simulink model "unicycle"  (R2024a)
settings: Solver=ode45  StartTime=0.0  StopTime=20.0  RelTol=1e-3
undefined symbols (not defined in the file): b_reference_point, damping_coefficient, damping_coefficient_nl, k1, k2, kp1, kp2, kp3, kp4, kv, kw, natural_frequency, natural_frequency_nl, radius, x1_dest, x2_dest, x3_dest
libraries: simulink x6, robotmobilelib x3
(part 1 of 2)
settings Model: Creator=leona  LastModifiedBy=meteh
settings SolverCC: ZeroCrossAlgorithm=Adaptive
settings DataIOCC: SaveFinalState=on  SaveFormat=StructureWithTime  SaveState=on  SignalLogging=off
settings DebuggingCC: IgnoredZcDiagnostic=none

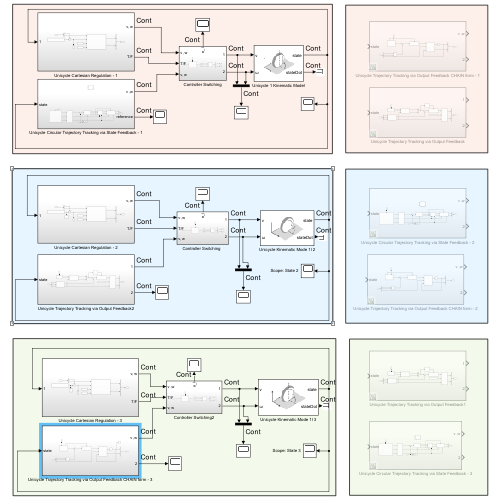
[thumbnail: Simulink's stored preview of the top-level diagram]
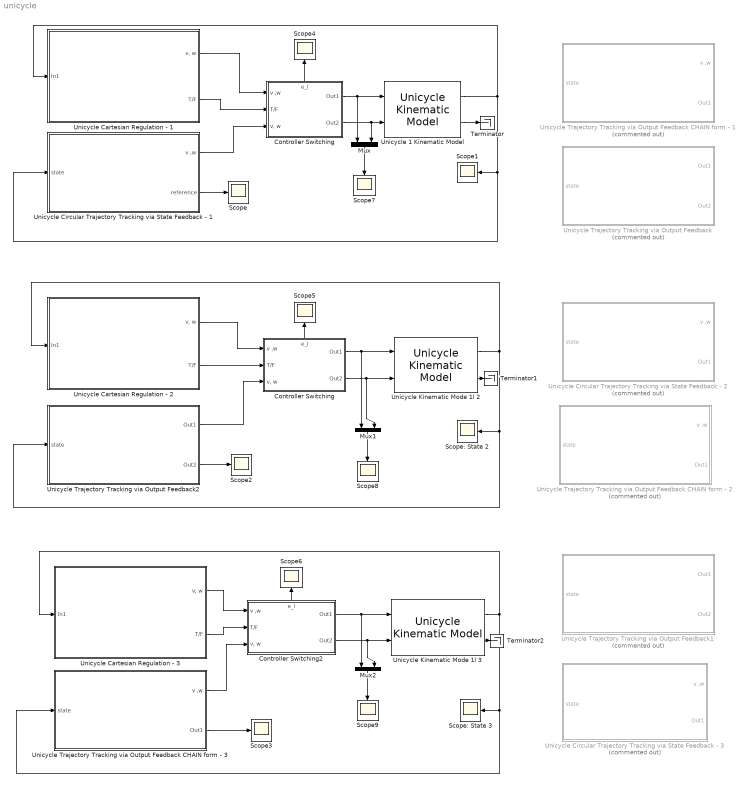
== system unicycle ==
  Controller Switching : Subsystem
      settings: PortSchema="{\"entries\":[{\"content\":{\"sides\":[{\"content\":{\"connectorIds\":[\"In1\",\"In2\",\"In3\"]},\"type\":\"ConnectorPlacement.EquallySpacedRectSide\",\"uuid\":\"584f21ea-dfd6-45f5-be40-b293bc8457b1\"},{\"content\":{\"connectorIds\":[\"Out1\",\"Out2\"],\"side\":\"RIGHT\"},\"type\":\"ConnectorPlacement.EquallySpacedRectSide\",\"uuid\":\"f9bf7ef9-3ae2-4892-b478-b0129d05cdbd\"},{\"content\":{\"connectorIds\":[\"Out3\"],\"side\":\"TOP\"},\"type\":\"ConnectorPlacement.EquallySpacedRectSide\",\"uuid\":\"62fa3bd1-cc21-4bdf-9148-7b9ede413ebd\"}]},\"type\":\"ConnectorPlacement.EquallySpacedConnector\",\"uuid\":\"adaa0c4e-8ae6-4cf2-baff-ed3c22a40f8d\"}],\"packageUris\":[\"http://schema.mathworks.com/mf0/Connector/R2020b\"],\"version\":\"1.0\"}"
  "Controller Switching  " : Subsystem
      settings: PortSchema="{\"entries\":[{\"content\":{\"sides\":[{\"content\":{\"connectorIds\":[\"In1\",\"In2\",\"In3\"]},\"type\":\"ConnectorPlacement.EquallySpacedRectSide\",\"uuid\":\"584f21ea-dfd6-45f5-be40-b293bc8457b1\"},{\"content\":{\"connectorIds\":[\"Out1\",\"Out2\"],\"side\":\"RIGHT\"},\"type\":\"ConnectorPlacement.EquallySpacedRectSide\",\"uuid\":\"f9bf7ef9-3ae2-4892-b478-b0129d05cdbd\"},{\"content\":{\"connectorIds\":[\"Out3\"],\"side\":\"TOP\"},\"type\":\"ConnectorPlacement.EquallySpacedRectSide\",\"uuid\":\"62fa3bd1-cc21-4bdf-9148-7b9ede413ebd\"}]},\"type\":\"ConnectorPlacement.EquallySpacedConnector\",\"uuid\":\"adaa0c4e-8ae6-4cf2-baff-ed3c22a40f8d\"}],\"packageUris\":[\"http://schema.mathworks.com/mf0/Connector/R2020b\"],\"version\":\"1.0\"}"
  Controller Switching2 : Subsystem
      settings: PortSchema="{\"entries\":[{\"content\":{\"sides\":[{\"content\":{\"connectorIds\":[\"In1\",\"In2\",\"In3\"]},\"type\":\"ConnectorPlacement.EquallySpacedRectSide\",\"uuid\":\"584f21ea-dfd6-45f5-be40-b293bc8457b1\"},{\"content\":{\"connectorIds\":[\"Out1\",\"Out2\"],\"side\":\"RIGHT\"},\"type\":\"ConnectorPlacement.EquallySpacedRectSide\",\"uuid\":\"f9bf7ef9-3ae2-4892-b478-b0129d05cdbd\"},{\"content\":{\"connectorIds\":[\"Out3\"],\"side\":\"TOP\"},\"type\":\"ConnectorPlacement.EquallySpacedRectSide\",\"uuid\":\"62fa3bd1-cc21-4bdf-9148-7b9ede413ebd\"}]},\"type\":\"ConnectorPlacement.EquallySpacedConnector\",\"uuid\":\"adaa0c4e-8ae6-4cf2-baff-ed3c22a40f8d\"}],\"packageUris\":[\"http://schema.mathworks.com/mf0/Connector/R2020b\"],\"version\":\"1.0\"}"
  Mux : Mux  Inputs=2
  Mux1 : Mux  Inputs=2
  Mux2 : Mux  Inputs=2
  Scope{,1..9} (10 alike) : Scope
  Scope: State 2 : Scope
  Scope: State 3 : Scope
  Terminator : Terminator
  Terminator1 : Terminator
  Terminator2 : Terminator
  Unicycle 1 Kinematic Model : robotmobilelib/Unicycle Kinematic Model  VehicleInputs=Vehicle Speed & Heading Angular Velocity  WheelRadius=wheel_radius  WheelSpeedRange=wheel_speed_range  InitialState=init_state_1  SimulateUsing=Interpreted execution
  Unicycle Cartesian Regulation - 1 : Subsystem
  Unicycle Cartesian Regulation - 2 : Subsystem
  Unicycle Cartesian Regulation - 3 : Subsystem
  Unicycle Circular Trajectory Tracking via State Feedback - 1 : Subsystem
  Unicycle Circular Trajectory Tracking via State Feedback - 2 : Subsystem  Commented=on
  Unicycle Circular Trajectory Tracking via State Feedback - 3 : Subsystem  Commented=on
  Unicycle Kinematic Mode 1l 2 : robotmobilelib/Unicycle Kinematic Model  VehicleInputs=Vehicle Speed & Heading Angular Velocity  WheelRadius=wheel_radius  WheelSpeedRange=wheel_speed_range  InitialState=init_state_2  SimulateUsing=Interpreted execution
  Unicycle Kinematic Mode 1l 3 : robotmobilelib/Unicycle Kinematic Model  VehicleInputs=Vehicle Speed & Heading Angular Velocity  WheelRadius=wheel_radius  WheelSpeedRange=wheel_speed_range  InitialState=init_state_3  SimulateUsing=Interpreted execution
  Unicycle Trajectory Tracking via Output Feedback : Subsystem  Commented=on
  Unicycle Trajectory Tracking via Output Feedback CHAIN form - 1 : Subsystem  Commented=on
  Unicycle Trajectory Tracking via Output Feedback CHAIN form - 2 : Subsystem  Commented=on
  Unicycle Trajectory Tracking via Output Feedback CHAIN form - 3 : Subsystem
  Unicycle Trajectory Tracking via Output Feedback1 : Subsystem  Commented=on
  Unicycle Trajectory Tracking via Output Feedback2 : Subsystem
  wires:
  Unicycle Cartesian Regulation - 1/1("v, w") -> Controller Switching/1(v ,w)
  Controller Switching/2(Out2) -> Mux/2, Unicycle 1 Kinematic Model/2
  Controller Switching/1(Out1) -> Unicycle 1 Kinematic Model/1, Mux/1
  Unicycle 1 Kinematic Model/1 -> Unicycle Cartesian Regulation - 1/1(In1), Unicycle Circular Trajectory Tracking via State Feedback - 1/1("state "), Scope1/1
  Unicycle Circular Trajectory Tracking via State Feedback - 1/1(v ,w) -> Controller Switching/3("v, w")
  Unicycle Cartesian Regulation - 1/2(T/F) -> Controller Switching/2(T/F)
  Unicycle Cartesian Regulation - 2/1("v, w") -> "Controller Switching  "/1(v ,w)
  Unicycle Cartesian Regulation - 2/2(T/F) -> "Controller Switching  "/2(T/F)
  Unicycle Trajectory Tracking via Output Feedback2/1(Out1) -> "Controller Switching  "/3("v, w")
  Unicycle Kinematic Mode 1l 2/2 -> Terminator1/1
  Unicycle Kinematic Mode 1l 2/1 -> Unicycle Cartesian Regulation - 2/1(In1), Unicycle Trajectory Tracking via Output Feedback2/1(state), Scope: State 2/1
  Controller Switching2/2(Out2) -> Unicycle Kinematic Mode 1l 3/2, Mux2/2
  Unicycle Kinematic Mode 1l 3/2 -> Terminator2/1
  Unicycle Kinematic Mode 1l 3/1 -> Unicycle Cartesian Regulation - 3/1(In1), Unicycle Trajectory Tracking via Output Feedback CHAIN form - 3/1(state), Scope: State 3/1
  Controller Switching2/1(Out1) -> Mux2/1, Unicycle Kinematic Mode 1l 3/1
  Unicycle 1 Kinematic Model/2 -> Terminator/1
  Unicycle Cartesian Regulation - 3/1("v, w") -> Controller Switching2/1(v ,w)
  Unicycle Cartesian Regulation - 3/2(T/F) -> Controller Switching2/2(T/F)
  Unicycle Trajectory Tracking via Output Feedback CHAIN form - 3/1(v ,w) -> Controller Switching2/3("v, w")
  Unicycle Circular Trajectory Tracking via State Feedback - 1/2(reference) -> Scope/1
  Unicycle Trajectory Tracking via Output Feedback2/2(Out2) -> Scope2/1
  Unicycle Trajectory Tracking via Output Feedback CHAIN form - 3/2(Out1) -> Scope3/1
  Controller Switching/3(e_l) -> Scope4/1
  "Controller Switching  "/3(e_l) -> Scope5/1
  Controller Switching2/3(e_l) -> Scope6/1
  Mux/1 -> Scope7/1
  Mux1/1 -> Scope8/1
  Mux2/1 -> Scope9/1
  "Controller Switching  "/1(Out1) -> Unicycle Kinematic Mode 1l 2/1, Mux1/1
  "Controller Switching  "/2(Out2) -> Mux1/2, Unicycle Kinematic Mode 1l 2/2

== system unicycle/Controller Switching ==
  v ,w : Inport
  T/F : Inport  Port=2
  "v, w" : Inport  Port=3
  Boolean Logic : Subsystem
      settings: PortSchema="{\"entries\":[{\"content\":{\"sides\":[{\"content\":{\"connectorIds\":[\"In1\"]},\"type\":\"ConnectorPlacement.EquallySpacedRectSide\",\"uuid\":\"34f08167-0350-4dbe-87ce-831ff9562b76\"},{\"content\":{\"connectorIds\":[\"Out1\"],\"side\":\"RIGHT\"},\"type\":\"ConnectorPlacement.EquallySpacedRectSide\",\"uuid\":\"220e97c4-e345-4de7-8cbd-23fec7576d43\"},{\"content\":{\"connectorIds\":[\"Out2\"],\"side\":\"TOP\"},\"type\":\"ConnectorPlacement.EquallySpacedRectSide\",\"uuid\":\"03b95ec6-4170-48da-8e0d-314706af41d0\"}]},\"type\":\"ConnectorPlacement.EquallySpacedConnector\",\"uuid\":\"155ce1e7-d9ad-489e-93e0-8e88a3bed561\"}],\"packageUris\":[\"http://schema.mathworks.com/mf0/Connector/R2020b\"],\"version\":\"1.0\"}"
  Demux1 : Demux  Outputs=2
  Switch1 : Switch  Criteria=u2 > Threshold  SaturateOnIntegerOverflow=off  InputSameDT=off
  Out1 : Outport
  Out2 : Outport  Port=2
  e_l : Outport  Port=3
  wires:
  Switch1/1 -> Demux1/1
  Demux1/2 -> Out2/1
  Demux1/1 -> Out1/1
  v ,w/1 -> Switch1/3
  "v, w"/1 -> Switch1/1
  Boolean Logic/1(Out1) -> Switch1/2
  T/F/1 -> Boolean Logic/1(e)
  Boolean Logic/2(e_l) -> e_l/1

== system unicycle/Controller Switching   ==
  v ,w : Inport
  T/F : Inport  Port=2
  "v, w" : Inport  Port=3
  Boolean Logic : Subsystem
      settings: PortSchema="{\"entries\":[{\"content\":{\"sides\":[{\"content\":{\"connectorIds\":[\"In1\"]},\"type\":\"ConnectorPlacement.EquallySpacedRectSide\",\"uuid\":\"34f08167-0350-4dbe-87ce-831ff9562b76\"},{\"content\":{\"connectorIds\":[\"Out1\"],\"side\":\"RIGHT\"},\"type\":\"ConnectorPlacement.EquallySpacedRectSide\",\"uuid\":\"220e97c4-e345-4de7-8cbd-23fec7576d43\"},{\"content\":{\"connectorIds\":[\"Out2\"],\"side\":\"TOP\"},\"type\":\"ConnectorPlacement.EquallySpacedRectSide\",\"uuid\":\"03b95ec6-4170-48da-8e0d-314706af41d0\"}]},\"type\":\"ConnectorPlacement.EquallySpacedConnector\",\"uuid\":\"155ce1e7-d9ad-489e-93e0-8e88a3bed561\"}],\"packageUris\":[\"http://schema.mathworks.com/mf0/Connector/R2020b\"],\"version\":\"1.0\"}"
  Demux1 : Demux  Outputs=2
  Switch1 : Switch  Criteria=u2 > Threshold  SaturateOnIntegerOverflow=off  InputSameDT=off
  Out1 : Outport
  Out2 : Outport  Port=2
  e_l : Outport  Port=3
  wires:
  Switch1/1 -> Demux1/1
  Demux1/2 -> Out2/1
  Demux1/1 -> Out1/1
  v ,w/1 -> Switch1/3
  "v, w"/1 -> Switch1/1
  Boolean Logic/1(Out1) -> Switch1/2
  T/F/1 -> Boolean Logic/1(e)
  Boolean Logic/2(e_l) -> e_l/1

== system unicycle/Controller Switching2 ==
  v ,w : Inport
  T/F : Inport  Port=2
  "v, w" : Inport  Port=3
  Boolean Logic : Subsystem
      settings: PortSchema="{\"entries\":[{\"content\":{\"sides\":[{\"content\":{\"connectorIds\":[\"In1\"]},\"type\":\"ConnectorPlacement.EquallySpacedRectSide\",\"uuid\":\"34f08167-0350-4dbe-87ce-831ff9562b76\"},{\"content\":{\"connectorIds\":[\"Out1\"],\"side\":\"RIGHT\"},\"type\":\"ConnectorPlacement.EquallySpacedRectSide\",\"uuid\":\"220e97c4-e345-4de7-8cbd-23fec7576d43\"},{\"content\":{\"connectorIds\":[\"Out2\"],\"side\":\"TOP\"},\"type\":\"ConnectorPlacement.EquallySpacedRectSide\",\"uuid\":\"03b95ec6-4170-48da-8e0d-314706af41d0\"}]},\"type\":\"ConnectorPlacement.EquallySpacedConnector\",\"uuid\":\"155ce1e7-d9ad-489e-93e0-8e88a3bed561\"}],\"packageUris\":[\"http://schema.mathworks.com/mf0/Connector/R2020b\"],\"version\":\"1.0\"}"
  Demux1 : Demux  Outputs=2
  Switch1 : Switch  Criteria=u2 > Threshold  SaturateOnIntegerOverflow=off  InputSameDT=off
  Out1 : Outport
  Out2 : Outport  Port=2
  e_l : Outport  Port=3
  wires:
  Switch1/1 -> Demux1/1
  Demux1/2 -> Out2/1
  Demux1/1 -> Out1/1
  v ,w/1 -> Switch1/3
  "v, w"/1 -> Switch1/1
  Boolean Logic/1(Out1) -> Switch1/2
  T/F/1 -> Boolean Logic/1(e)
  Boolean Logic/2(e_l) -> e_l/1

== system unicycle/Unicycle Cartesian Regulation - 1 ==
  In1 : Inport
  Constant2 : Constant  Value=kv
  Constant3 : Constant  Value=kw
  Demux2 : Demux  Outputs=2
  Mux1 : Mux  Inputs=2
  Regulation Controller1 : MATLAB Function  TreatAsAtomicUnit=on
  Rendez-vous destination : Constant  Value=[x1_dest(1,1), x1_dest(1,2)]
  Sum3 : Sum  Inputs=-+|
  "v, w" : Outport
  T/F : Outport  Port=2
  wires:
  Sum3/1 -> Regulation Controller1/2(e), T/F/1
  Regulation Controller1/1(v) -> Mux1/1
  Regulation Controller1/2(w) -> Mux1/2
  Mux1/1 -> "v, w"/1
  In1/1 -> Demux2/1
  Demux2/1 -> Sum3/1
  Rendez-vous destination/1 -> Sum3/2
  Demux2/2 -> Regulation Controller1/1(theta)
  Constant2/1 -> Regulation Controller1/3(kv)
  Constant3/1 -> Regulation Controller1/4(kw)

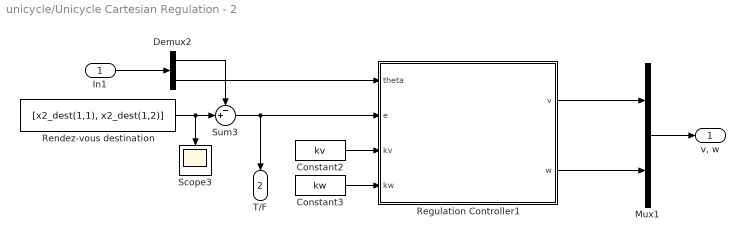
== system unicycle/Unicycle Cartesian Regulation - 2 ==
  In1 : Inport
  Constant2 : Constant  Value=kv
  Constant3 : Constant  Value=kw
  Demux2 : Demux  Outputs=2
  Mux1 : Mux  Inputs=2
  Regulation Controller1 : MATLAB Function  TreatAsAtomicUnit=on
  Rendez-vous destination : Constant  Value=[x2_dest(1,1), x2_dest(1,2)]
  Scope3 : Scope
  Sum3 : Sum  Inputs=-+|
  "v, w" : Outport
  T/F : Outport  Port=2
  wires:
  Sum3/1 -> Regulation Controller1/2(e), T/F/1
  Regulation Controller1/1(v) -> Mux1/1
  Regulation Controller1/2(w) -> Mux1/2
  Mux1/1 -> "v, w"/1
  In1/1 -> Demux2/1
  Demux2/1 -> Sum3/1
  Rendez-vous destination/1 -> Sum3/2, Scope3/1
  Demux2/2 -> Regulation Controller1/1(theta)
  Constant2/1 -> Regulation Controller1/3(kv)
  Constant3/1 -> Regulation Controller1/4(kw)

== system unicycle/Unicycle Cartesian Regulation - 3 ==
  In1 : Inport
  Constant2 : Constant  Value=kv
  Constant3 : Constant  Value=kw
  Demux2 : Demux  Outputs=2
  Mux1 : Mux  Inputs=2
  Regulation Controller1 : MATLAB Function  TreatAsAtomicUnit=on
  Rendez-vous destination : Constant  Value=[x3_dest(1,1), x3_dest(1,2)]
  Scope3 : Scope
  Sum3 : Sum  Inputs=-+|
  "v, w" : Outport
  T/F : Outport  Port=2
  wires:
  Sum3/1 -> Regulation Controller1/2(e), T/F/1
  Regulation Controller1/1(v) -> Mux1/1
  Regulation Controller1/2(w) -> Mux1/2
  Mux1/1 -> "v, w"/1
  In1/1 -> Demux2/1
  Demux2/1 -> Sum3/1
  Rendez-vous destination/1 -> Sum3/2, Scope3/1
  Demux2/2 -> Regulation Controller1/1(theta)
  Constant2/1 -> Regulation Controller1/3(kv)
  Constant3/1 -> Regulation Controller1/4(kw)

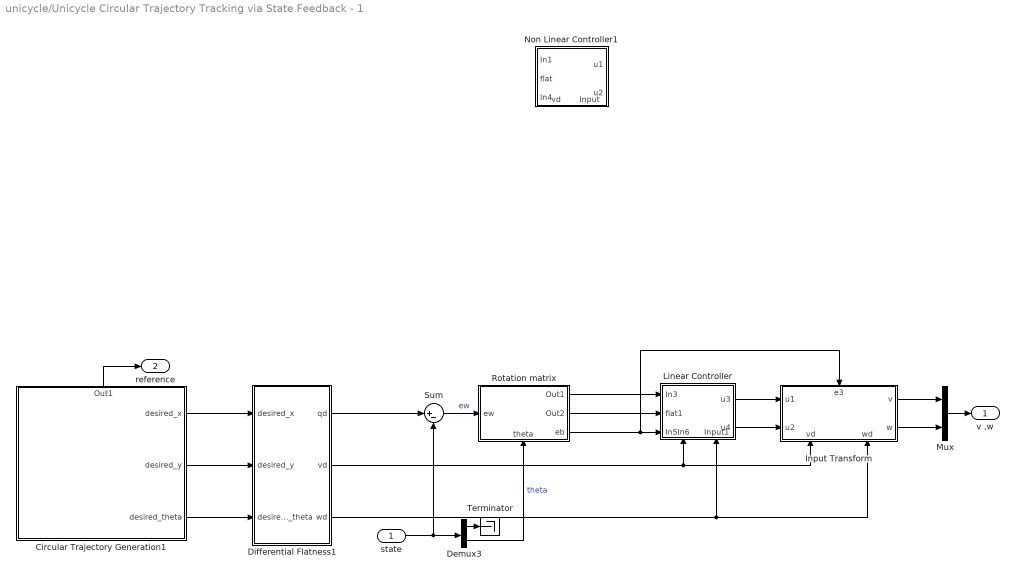
== system unicycle/Unicycle Circular Trajectory Tracking via State Feedback - 1 ==
  "state " : Inport
  Circular Trajectory Generation1 : Subsystem
      settings: PortSchema="{\"entries\":[{\"content\":{\"sides\":[{\"content\":{},\"type\":\"ConnectorPlacement.EquallySpacedRectSide\",\"uuid\":\"3fbc7189-acaa-4619-a293-0370d4e72fe2\"},{\"content\":{\"connectorIds\":[\"Out1\",\"Out2\",\"Out3\"],\"side\":\"RIGHT\"},\"type\":\"ConnectorPlacement.EquallySpacedRectSide\",\"uuid\":\"ce8f3bde-3ad4-4866-8ed9-b77e72e9e477\"},{\"content\":{\"connectorIds\":[\"Out4\"],\"side\":\"TOP\"},\"type\":\"ConnectorPlacement.EquallySpacedRectSide\",\"uuid\":\"5afa6f18-5aff-4e43-8316-9d22777d6d8b\"}]},\"type\":\"ConnectorPlacement.EquallySpacedConnector\",\"uuid\":\"0a9ab007-6c25-4113-bd09-eb536dbf5551\"}],\"packageUris\":[\"http://schema.mathworks.com/mf0/Connector/R2020b\"],\"version\":\"1.0\"}"
  Demux3 : Demux  Outputs=2
  Differential Flatness1 : Subsystem
  Input Transform : Subsystem
      settings: PortSchema="{\"entries\":[{\"content\":{\"sides\":[{\"content\":{\"connectorIds\":[\"In1\",\"In2\"]},\"type\":\"ConnectorPlacement.EquallySpacedRectSide\",\"uuid\":\"4380a799-56bd-42fa-b7eb-8f0915c9014b\"},{\"content\":{\"connectorIds\":[\"Out1\",\"Out2\"],\"side\":\"RIGHT\"},\"type\":\"ConnectorPlacement.EquallySpacedRectSide\",\"uuid\":\"97586fd2-c031-459c-92a6-bfbe946839f3\"},{\"content\":{\"connectorIds\":[\"In3\"],\"side\":\"TOP\"},\"type\":\"ConnectorPlacement.EquallySpacedRectSide\",\"uuid\":\"9290dd6f-8297-418b-8b82-c5c2ebc9030b\"},{\"content\":{\"connectorIds\":[\"In4\",\"In5\"],\"side\":\"BOTTOM\"},\"type\":\"ConnectorPlacement.EquallySpacedRectSide\",\"uuid\":\"808db643-f3c8-472e-94d3-d65694c039e0\"}]},\"type\":\"ConnectorPlacement.EquallySpacedConnector\",\"uuid\":\"008e5a81-0e40-4b3a-a5f3-e29ef3b642db\"}],\"packageUris\":[\"http://schema.mathworks.com/mf0/Connector/R2020b\"],\"version\":\"1.0\"}"
  Linear Controller : Subsystem
      settings: PortSchema="{\"entries\":[{\"content\":{\"sides\":[{\"content\":{},\"type\":\"ConnectorPlacement.EquallySpacedRectSide\",\"uuid\":\"355dd5aa-d78b-48af-8d08-54ec3378b437\"},{\"content\":{\"connectorIds\":[\"In4\",\"In5\"],\"side\":\"RIGHT\"},\"type\":\"ConnectorPlacement.EquallySpacedRectSide\",\"uuid\":\"4abc5e76-df33-4792-8900-ee46a2dcc207\"},{\"content\":{\"connectorIds\":[\"Out1\",\"Out2\"],\"side\":\"TOP\"},\"type\":\"ConnectorPlacement.EquallySpacedRectSide\",\"uuid\":\"520b05a2-b812-4ca4-b90c-01a128f1edcc\"},{\"content\":{\"connectorIds\":[\"In1\",\"In2\",\"In3\"],\"side\":\"BOTTOM\"},\"type\":\"ConnectorPlacement.EquallySpacedRectSide\",\"uuid\":\"7b1db8d6-e255-4c64-80bc-17cc7e8073d1\"}]},\"type\":\"ConnectorPlacement.EquallySpacedConnector\",\"uuid\":\"a570cf3a-e792-4caa-b5b1-65826e704bdc\"}],\"packageUris\":[\"http://schema.mathworks.com/mf0/Connector/R2020b\"],\"version\":\"1.0\"}"
  Mux : Mux  Inputs=2
  Non Linear Controller1 : Subsystem
      settings: PortSchema="{\"entries\":[{\"content\":{\"sides\":[{\"content\":{\"connectorIds\":[\"In1\",\"In2\",\"In3\"]},\"type\":\"ConnectorPlacement.EquallySpacedRectSide\",\"uuid\":\"355dd5aa-d78b-48af-8d08-54ec3378b437\"},{\"content\":{\"connectorIds\":[\"Out1\",\"Out2\"],\"side\":\"RIGHT\"},\"type\":\"ConnectorPlacement.EquallySpacedRectSide\",\"uuid\":\"4abc5e76-df33-4792-8900-ee46a2dcc207\"},{\"content\":{\"side\":\"TOP\"},\"type\":\"ConnectorPlacement.EquallySpacedRectSide\",\"uuid\":\"520b05a2-b812-4ca4-b90c-01a128f1edcc\"},{\"content\":{\"connectorIds\":[\"In4\",\"In5\"],\"side\":\"BOTTOM\"},\"type\":\"ConnectorPlacement.EquallySpacedRectSide\",\"uuid\":\"7b1db8d6-e255-4c64-80bc-17cc7e8073d1\"}]},\"type\":\"ConnectorPlacement.EquallySpacedConnector\",\"uuid\":\"a570cf3a-e792-4caa-b5b1-65826e704bdc\"}],\"packageUris\":[\"http://schema.mathworks.com/mf0/Connector/R2020b\"],\"version\":\"1.0\"}"
  Rotation matrix : Subsystem
      settings: PortSchema="{\"entries\":[{\"content\":{\"sides\":[{\"content\":{\"connectorIds\":[\"In1\"]},\"type\":\"ConnectorPlacement.EquallySpacedRectSide\",\"uuid\":\"c80c5426-0069-418a-be1e-050f85102122\"},{\"content\":{\"connectorIds\":[\"Out1\",\"Out2\",\"Out3\"],\"side\":\"RIGHT\"},\"type\":\"ConnectorPlacement.EquallySpacedRectSide\",\"uuid\":\"f8dc66be-8604-4f98-b9fe-fa15c49770bc\"},{\"content\":{\"side\":\"TOP\"},\"type\":\"ConnectorPlacement.EquallySpacedRectSide\",\"uuid\":\"c5b1bfab-7e11-40da-b9ae-0f329f8970ce\"},{\"content\":{\"connectorIds\":[\"In2\"],\"side\":\"BOTTOM\"},\"type\":\"ConnectorPlacement.EquallySpacedRectSide\",\"uuid\":\"007620ed-2c8f-4927-b7e7-dbc9138b761c\"}]},\"type\":\"ConnectorPlacement.EquallySpacedConnector\",\"uuid\":\"efc411d4-2e62-4ef2-9268-9fb7a97f0e7c\"}],\"packageUris\":[\"http://schema.mathworks.com/mf0/Connector/R2020b\"],\"version\":\"1.0\"}"
  Sum : Sum  Inputs=|+-
  Terminator : Terminator
  v ,w : Outport
  reference : Outport  Port=2
  wires:
  Linear Controller/1(u3) -> Input Transform/1(u1)
  Linear Controller/2(u4) -> Input Transform/2(u2)
  Differential Flatness1/3(wd) -> Linear Controller/4(Input1), Input Transform/5(wd)
  Input Transform/1(v) -> Mux/1
  Differential Flatness1/2(vd) -> Linear Controller/5(In6), Input Transform/4(vd)
  Demux3/2 -> Rotation matrix/2(theta)  "theta"
  Differential Flatness1/1(qd) -> Sum/1
  Rotation matrix/1(Out1) -> Linear Controller/1(In3)
  Sum/1 -> Rotation matrix/1(ew)  "ew"
  Input Transform/2(w) -> Mux/2
  "state "/1 -> Demux3/1, Sum/2
  Rotation matrix/3(eb) -> Linear Controller/3(In5), Input Transform/3(e3)
  Rotation matrix/2(Out2) -> Linear Controller/2(flat1)
  Mux/1 -> v ,w/1
  Circular Trajectory Generation1/2(desired_y) -> Differential Flatness1/2(desired_y)
  Circular Trajectory Generation1/1(desired_x) -> Differential Flatness1/1(desired_x)
  Circular Trajectory Generation1/3(desired_theta) -> Differential Flatness1/3(desired_theta)
  Demux3/1 -> Terminator/1
  Circular Trajectory Generation1/4(Out1) -> reference/1

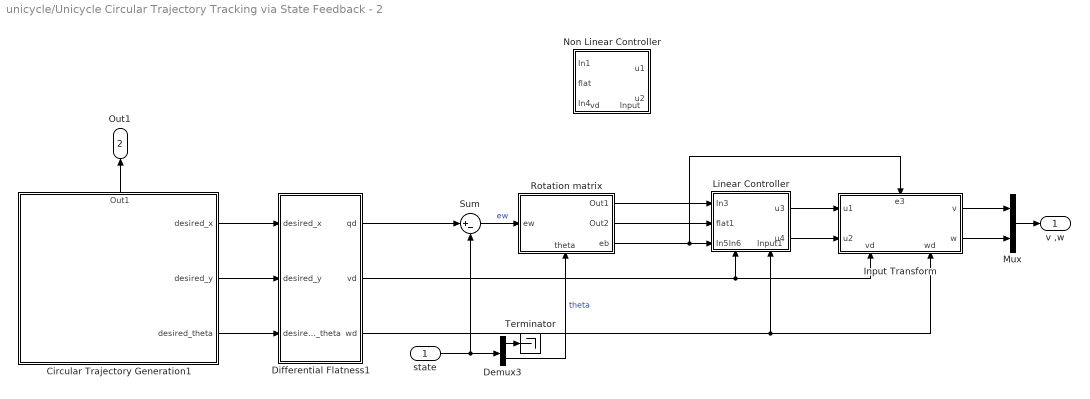
== system unicycle/Unicycle Circular Trajectory Tracking via State Feedback - 2 ==
  "state " : Inport
  Circular Trajectory Generation1 : Subsystem
      settings: PortSchema="{\"entries\":[{\"content\":{\"sides\":[{\"content\":{},\"type\":\"ConnectorPlacement.EquallySpacedRectSide\",\"uuid\":\"7eb2aa46-4d8f-40e4-84eb-88ddc260fd26\"},{\"content\":{\"connectorIds\":[\"Out1\",\"Out2\",\"Out3\"],\"side\":\"RIGHT\"},\"type\":\"ConnectorPlacement.EquallySpacedRectSide\",\"uuid\":\"c61c70de-cb1b-4693-a19f-0935ee593969\"},{\"content\":{\"connectorIds\":[\"Out4\"],\"side\":\"TOP\"},\"type\":\"ConnectorPlacement.EquallySpacedRectSide\",\"uuid\":\"a1bb1060-a0e1-4ec9-871f-7f02f1bdb938\"}]},\"type\":\"ConnectorPlacement.EquallySpacedConnector\",\"uuid\":\"5dd701f6-f55e-4dcb-a175-ac66dc826cad\"}],\"packageUris\":[\"http://schema.mathworks.com/mf0/Connector/R2020b\"],\"version\":\"1.0\"}"
  Demux3 : Demux  Outputs=2
  Differential Flatness1 : Subsystem
  Input Transform : Subsystem
      settings: PortSchema="{\"entries\":[{\"content\":{\"sides\":[{\"content\":{\"connectorIds\":[\"In1\",\"In2\"]},\"type\":\"ConnectorPlacement.EquallySpacedRectSide\",\"uuid\":\"4380a799-56bd-42fa-b7eb-8f0915c9014b\"},{\"content\":{\"connectorIds\":[\"Out1\",\"Out2\"],\"side\":\"RIGHT\"},\"type\":\"ConnectorPlacement.EquallySpacedRectSide\",\"uuid\":\"97586fd2-c031-459c-92a6-bfbe946839f3\"},{\"content\":{\"connectorIds\":[\"In3\"],\"side\":\"TOP\"},\"type\":\"ConnectorPlacement.EquallySpacedRectSide\",\"uuid\":\"9290dd6f-8297-418b-8b82-c5c2ebc9030b\"},{\"content\":{\"connectorIds\":[\"In4\",\"In5\"],\"side\":\"BOTTOM\"},\"type\":\"ConnectorPlacement.EquallySpacedRectSide\",\"uuid\":\"808db643-f3c8-472e-94d3-d65694c039e0\"}]},\"type\":\"ConnectorPlacement.EquallySpacedConnector\",\"uuid\":\"008e5a81-0e40-4b3a-a5f3-e29ef3b642db\"}],\"packageUris\":[\"http://schema.mathworks.com/mf0/Connector/R2020b\"],\"version\":\"1.0\"}"
  Linear Controller : Subsystem
      settings: PortSchema="{\"entries\":[{\"content\":{\"sides\":[{\"content\":{},\"type\":\"ConnectorPlacement.EquallySpacedRectSide\",\"uuid\":\"355dd5aa-d78b-48af-8d08-54ec3378b437\"},{\"content\":{\"connectorIds\":[\"In4\",\"In5\"],\"side\":\"RIGHT\"},\"type\":\"ConnectorPlacement.EquallySpacedRectSide\",\"uuid\":\"4abc5e76-df33-4792-8900-ee46a2dcc207\"},{\"content\":{\"connectorIds\":[\"Out1\",\"Out2\"],\"side\":\"TOP\"},\"type\":\"ConnectorPlacement.EquallySpacedRectSide\",\"uuid\":\"520b05a2-b812-4ca4-b90c-01a128f1edcc\"},{\"content\":{\"connectorIds\":[\"In1\",\"In2\",\"In3\"],\"side\":\"BOTTOM\"},\"type\":\"ConnectorPlacement.EquallySpacedRectSide\",\"uuid\":\"7b1db8d6-e255-4c64-80bc-17cc7e8073d1\"}]},\"type\":\"ConnectorPlacement.EquallySpacedConnector\",\"uuid\":\"a570cf3a-e792-4caa-b5b1-65826e704bdc\"}],\"packageUris\":[\"http://schema.mathworks.com/mf0/Connector/R2020b\"],\"version\":\"1.0\"}"
  Mux : Mux  Inputs=2
  Non Linear Controller : Subsystem
      settings: PortSchema="{\"entries\":[{\"content\":{\"sides\":[{\"content\":{\"connectorIds\":[\"In1\",\"In2\",\"In3\"]},\"type\":\"ConnectorPlacement.EquallySpacedRectSide\",\"uuid\":\"355dd5aa-d78b-48af-8d08-54ec3378b437\"},{\"content\":{\"connectorIds\":[\"Out1\",\"Out2\"],\"side\":\"RIGHT\"},\"type\":\"ConnectorPlacement.EquallySpacedRectSide\",\"uuid\":\"4abc5e76-df33-4792-8900-ee46a2dcc207\"},{\"content\":{\"side\":\"TOP\"},\"type\":\"ConnectorPlacement.EquallySpacedRectSide\",\"uuid\":\"520b05a2-b812-4ca4-b90c-01a128f1edcc\"},{\"content\":{\"connectorIds\":[\"In4\",\"In5\"],\"side\":\"BOTTOM\"},\"type\":\"ConnectorPlacement.EquallySpacedRectSide\",\"uuid\":\"7b1db8d6-e255-4c64-80bc-17cc7e8073d1\"}]},\"type\":\"ConnectorPlacement.EquallySpacedConnector\",\"uuid\":\"a570cf3a-e792-4caa-b5b1-65826e704bdc\"}],\"packageUris\":[\"http://schema.mathworks.com/mf0/Connector/R2020b\"],\"version\":\"1.0\"}"
  Rotation matrix : Subsystem
      settings: PortSchema="{\"entries\":[{\"content\":{\"sides\":[{\"content\":{\"connectorIds\":[\"In1\"]},\"type\":\"ConnectorPlacement.EquallySpacedRectSide\",\"uuid\":\"c80c5426-0069-418a-be1e-050f85102122\"},{\"content\":{\"connectorIds\":[\"Out1\",\"Out2\",\"Out3\"],\"side\":\"RIGHT\"},\"type\":\"ConnectorPlacement.EquallySpacedRectSide\",\"uuid\":\"f8dc66be-8604-4f98-b9fe-fa15c49770bc\"},{\"content\":{\"side\":\"TOP\"},\"type\":\"ConnectorPlacement.EquallySpacedRectSide\",\"uuid\":\"c5b1bfab-7e11-40da-b9ae-0f329f8970ce\"},{\"content\":{\"connectorIds\":[\"In2\"],\"side\":\"BOTTOM\"},\"type\":\"ConnectorPlacement.EquallySpacedRectSide\",\"uuid\":\"007620ed-2c8f-4927-b7e7-dbc9138b761c\"}]},\"type\":\"ConnectorPlacement.EquallySpacedConnector\",\"uuid\":\"efc411d4-2e62-4ef2-9268-9fb7a97f0e7c\"}],\"packageUris\":[\"http://schema.mathworks.com/mf0/Connector/R2020b\"],\"version\":\"1.0\"}"
  Sum : Sum  Inputs=|+-
  Terminator : Terminator
  v ,w : Outport
  Out1 : Outport  Port=2
  wires:
  Linear Controller/1(u3) -> Input Transform/1(u1)
  Linear Controller/2(u4) -> Input Transform/2(u2)
  Differential Flatness1/3(wd) -> Linear Controller/4(Input1), Input Transform/5(wd)
  Input Transform/1(v) -> Mux/1
  Differential Flatness1/2(vd) -> Linear Controller/5(In6), Input Transform/4(vd)
  Demux3/2 -> Rotation matrix/2(theta)  "theta"
  Differential Flatness1/1(qd) -> Sum/1
  Rotation matrix/1(Out1) -> Linear Controller/1(In3)
  Sum/1 -> Rotation matrix/1(ew)  "ew"
  Input Transform/2(w) -> Mux/2
  "state "/1 -> Demux3/1, Sum/2
  Rotation matrix/3(eb) -> Linear Controller/3(In5), Input Transform/3(e3)
  Rotation matrix/2(Out2) -> Linear Controller/2(flat1)
  Mux/1 -> v ,w/1
  Circular Trajectory Generation1/2(desired_y) -> Differential Flatness1/2(desired_y)
  Circular Trajectory Generation1/1(desired_x) -> Differential Flatness1/1(desired_x)
  Circular Trajectory Generation1/3(desired_theta) -> Differential Flatness1/3(desired_theta)
  Demux3/1 -> Terminator/1
  Circular Trajectory Generation1/4(Out1) -> Out1/1

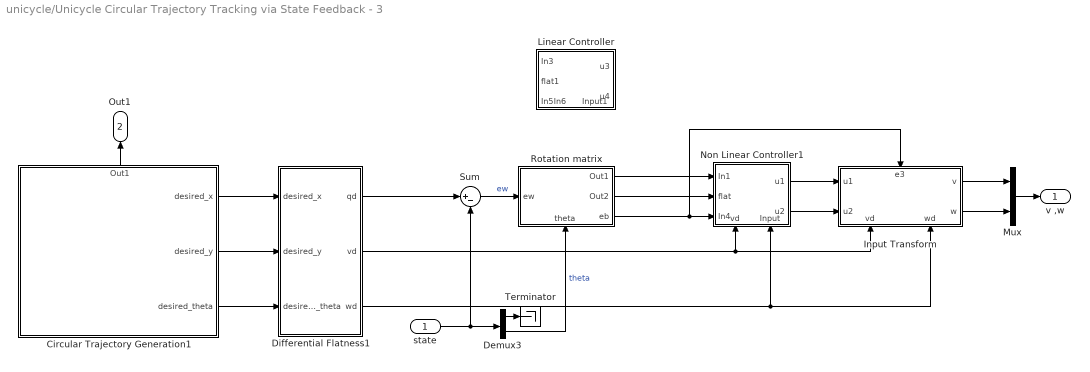
== system unicycle/Unicycle Circular Trajectory Tracking via State Feedback - 3 ==
  "state " : Inport
  Circular Trajectory Generation1 : Subsystem
      settings: PortSchema="{\"entries\":[{\"content\":{\"sides\":[{\"content\":{},\"type\":\"ConnectorPlacement.EquallySpacedRectSide\",\"uuid\":\"7eb2aa46-4d8f-40e4-84eb-88ddc260fd26\"},{\"content\":{\"connectorIds\":[\"Out1\",\"Out2\",\"Out3\"],\"side\":\"RIGHT\"},\"type\":\"ConnectorPlacement.EquallySpacedRectSide\",\"uuid\":\"c61c70de-cb1b-4693-a19f-0935ee593969\"},{\"content\":{\"connectorIds\":[\"Out4\"],\"side\":\"TOP\"},\"type\":\"ConnectorPlacement.EquallySpacedRectSide\",\"uuid\":\"a1bb1060-a0e1-4ec9-871f-7f02f1bdb938\"}]},\"type\":\"ConnectorPlacement.EquallySpacedConnector\",\"uuid\":\"5dd701f6-f55e-4dcb-a175-ac66dc826cad\"}],\"packageUris\":[\"http://schema.mathworks.com/mf0/Connector/R2020b\"],\"version\":\"1.0\"}"
  Demux3 : Demux  Outputs=2
  Differential Flatness1 : Subsystem
  Input Transform : Subsystem
      settings: PortSchema="{\"entries\":[{\"content\":{\"sides\":[{\"content\":{\"connectorIds\":[\"In1\",\"In2\"]},\"type\":\"ConnectorPlacement.EquallySpacedRectSide\",\"uuid\":\"4380a799-56bd-42fa-b7eb-8f0915c9014b\"},{\"content\":{\"connectorIds\":[\"Out1\",\"Out2\"],\"side\":\"RIGHT\"},\"type\":\"ConnectorPlacement.EquallySpacedRectSide\",\"uuid\":\"97586fd2-c031-459c-92a6-bfbe946839f3\"},{\"content\":{\"connectorIds\":[\"In3\"],\"side\":\"TOP\"},\"type\":\"ConnectorPlacement.EquallySpacedRectSide\",\"uuid\":\"9290dd6f-8297-418b-8b82-c5c2ebc9030b\"},{\"content\":{\"connectorIds\":[\"In4\",\"In5\"],\"side\":\"BOTTOM\"},\"type\":\"ConnectorPlacement.EquallySpacedRectSide\",\"uuid\":\"808db643-f3c8-472e-94d3-d65694c039e0\"}]},\"type\":\"ConnectorPlacement.EquallySpacedConnector\",\"uuid\":\"008e5a81-0e40-4b3a-a5f3-e29ef3b642db\"}],\"packageUris\":[\"http://schema.mathworks.com/mf0/Connector/R2020b\"],\"version\":\"1.0\"}"
  Linear Controller : Subsystem
      settings: PortSchema="{\"entries\":[{\"content\":{\"sides\":[{\"content\":{},\"type\":\"ConnectorPlacement.EquallySpacedRectSide\",\"uuid\":\"355dd5aa-d78b-48af-8d08-54ec3378b437\"},{\"content\":{\"connectorIds\":[\"In4\",\"In5\"],\"side\":\"RIGHT\"},\"type\":\"ConnectorPlacement.EquallySpacedRectSide\",\"uuid\":\"4abc5e76-df33-4792-8900-ee46a2dcc207\"},{\"content\":{\"connectorIds\":[\"Out1\",\"Out2\"],\"side\":\"TOP\"},\"type\":\"ConnectorPlacement.EquallySpacedRectSide\",\"uuid\":\"520b05a2-b812-4ca4-b90c-01a128f1edcc\"},{\"content\":{\"connectorIds\":[\"In1\",\"In2\",\"In3\"],\"side\":\"BOTTOM\"},\"type\":\"ConnectorPlacement.EquallySpacedRectSide\",\"uuid\":\"7b1db8d6-e255-4c64-80bc-17cc7e8073d1\"}]},\"type\":\"ConnectorPlacement.EquallySpacedConnector\",\"uuid\":\"a570cf3a-e792-4caa-b5b1-65826e704bdc\"}],\"packageUris\":[\"http://schema.mathworks.com/mf0/Connector/R2020b\"],\"version\":\"1.0\"}"
  Mux : Mux  Inputs=2
  Non Linear Controller1 : Subsystem
      settings: PortSchema="{\"entries\":[{\"content\":{\"sides\":[{\"content\":{\"connectorIds\":[\"In1\",\"In2\",\"In3\"]},\"type\":\"ConnectorPlacement.EquallySpacedRectSide\",\"uuid\":\"355dd5aa-d78b-48af-8d08-54ec3378b437\"},{\"content\":{\"connectorIds\":[\"Out1\",\"Out2\"],\"side\":\"RIGHT\"},\"type\":\"ConnectorPlacement.EquallySpacedRectSide\",\"uuid\":\"4abc5e76-df33-4792-8900-ee46a2dcc207\"},{\"content\":{\"side\":\"TOP\"},\"type\":\"ConnectorPlacement.EquallySpacedRectSide\",\"uuid\":\"520b05a2-b812-4ca4-b90c-01a128f1edcc\"},{\"content\":{\"connectorIds\":[\"In4\",\"In5\"],\"side\":\"BOTTOM\"},\"type\":\"ConnectorPlacement.EquallySpacedRectSide\",\"uuid\":\"7b1db8d6-e255-4c64-80bc-17cc7e8073d1\"}]},\"type\":\"ConnectorPlacement.EquallySpacedConnector\",\"uuid\":\"a570cf3a-e792-4caa-b5b1-65826e704bdc\"}],\"packageUris\":[\"http://schema.mathworks.com/mf0/Connector/R2020b\"],\"version\":\"1.0\"}"
  Rotation matrix : Subsystem
      settings: PortSchema="{\"entries\":[{\"content\":{\"sides\":[{\"content\":{\"connectorIds\":[\"In1\"]},\"type\":\"ConnectorPlacement.EquallySpacedRectSide\",\"uuid\":\"c80c5426-0069-418a-be1e-050f85102122\"},{\"content\":{\"connectorIds\":[\"Out1\",\"Out2\",\"Out3\"],\"side\":\"RIGHT\"},\"type\":\"ConnectorPlacement.EquallySpacedRectSide\",\"uuid\":\"f8dc66be-8604-4f98-b9fe-fa15c49770bc\"},{\"content\":{\"side\":\"TOP\"},\"type\":\"ConnectorPlacement.EquallySpacedRectSide\",\"uuid\":\"c5b1bfab-7e11-40da-b9ae-0f329f8970ce\"},{\"content\":{\"connectorIds\":[\"In2\"],\"side\":\"BOTTOM\"},\"type\":\"ConnectorPlacement.EquallySpacedRectSide\",\"uuid\":\"007620ed-2c8f-4927-b7e7-dbc9138b761c\"}]},\"type\":\"ConnectorPlacement.EquallySpacedConnector\",\"uuid\":\"efc411d4-2e62-4ef2-9268-9fb7a97f0e7c\"}],\"packageUris\":[\"http://schema.mathworks.com/mf0/Connector/R2020b\"],\"version\":\"1.0\"}"
  Sum : Sum  Inputs=|+-
  Terminator : Terminator
  v ,w : Outport
  Out1 : Outport  Port=2
  wires:
  Mux/1 -> v ,w/1
  Demux3/1 -> Terminator/1
  Circular Trajectory Generation1/1(desired_x) -> Differential Flatness1/1(desired_x)
  Circular Trajectory Generation1/3(desired_theta) -> Differential Flatness1/3(desired_theta)
  Rotation matrix/3(eb) -> Non Linear Controller1/3(In4), Input Transform/3(e3)
  Sum/1 -> Rotation matrix/1(ew)  "ew"
  Non Linear Controller1/1(u1) -> Input Transform/1(u1)
  Circular Trajectory Generation1/2(desired_y) -> Differential Flatness1/2(desired_y)
  Input Transform/2(w) -> Mux/2
  "state "/1 -> Demux3/1, Sum/2
  Rotation matrix/2(Out2) -> Non Linear Controller1/2(flat)
  Rotation matrix/1(Out1) -> Non Linear Controller1/1(In1)
  Differential Flatness1/2(vd) -> Non Linear Controller1/4(vd), Input Transform/4(vd)
  Differential Flatness1/3(wd) -> Non Linear Controller1/5(Input), Input Transform/5(wd)
  Differential Flatness1/1(qd) -> Sum/1
  Input Transform/1(v) -> Mux/1
  Non Linear Controller1/2(u2) -> Input Transform/2(u2)
  Demux3/2 -> Rotation matrix/2(theta)  "theta"
  Circular Trajectory Generation1/4(Out1) -> Out1/1

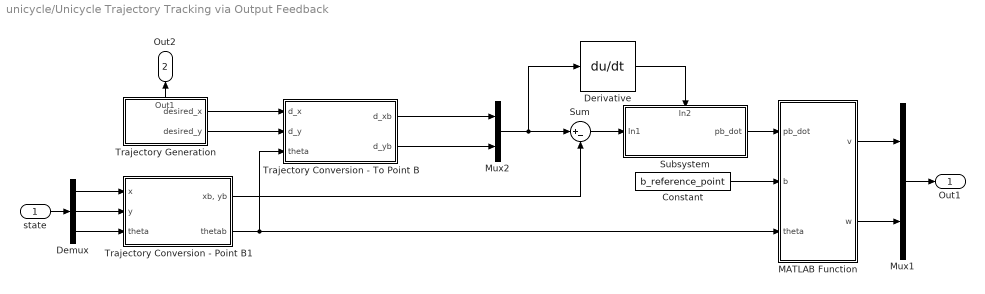
== system unicycle/Unicycle Trajectory Tracking via Output Feedback ==
  state : Inport
  Constant : Constant  Value=b_reference_point
  Demux : Demux  Outputs=3
  Derivative : Derivative
  MATLAB Function : MATLAB Function  TreatAsAtomicUnit=on
  Mux1 : Mux  Inputs=2
  Mux2 : Mux  Inputs=2
  Subsystem : Subsystem
      settings: PortSchema="{\"entries\":[{\"content\":{\"sides\":[{\"content\":{\"connectorIds\":[\"In1\"]},\"type\":\"ConnectorPlacement.EquallySpacedRectSide\",\"uuid\":\"e1edc101-a826-4003-ad08-df84a6d82578\"},{\"content\":{\"connectorIds\":[\"Out1\"],\"side\":\"RIGHT\"},\"type\":\"ConnectorPlacement.EquallySpacedRectSide\",\"uuid\":\"f1ed9078-3db7-4a0b-b785-0b08f9ba65fc\"},{\"content\":{\"connectorIds\":[\"In2\"],\"side\":\"TOP\"},\"type\":\"ConnectorPlacement.EquallySpacedRectSide\",\"uuid\":\"e7fa8122-daf7-4fc2-869b-ae0dcfffd8f2\"}]},\"type\":\"ConnectorPlacement.EquallySpacedConnector\",\"uuid\":\"a8720b8b-968d-49c2-bed5-00f70d36dfc2\"}],\"packageUris\":[\"http://schema.mathworks.com/mf0/Connector/R2020b\"],\"version\":\"1.0\"}"
  Sum : Sum  Inputs=|+-
  Trajectory Conversion - Point B1 : Subsystem
  Trajectory Conversion - To Point B : Subsystem
  Trajectory Generation : Subsystem
      settings: PortSchema="{\"entries\":[{\"content\":{\"sides\":[{\"content\":{},\"type\":\"ConnectorPlacement.EquallySpacedRectSide\",\"uuid\":\"27f935c9-4c91-4862-b00f-49430b536ba0\"},{\"content\":{\"connectorIds\":[\"Out1\",\"Out2\"],\"side\":\"RIGHT\"},\"type\":\"ConnectorPlacement.EquallySpacedRectSide\",\"uuid\":\"fd268e79-917c-4566-a618-4e3d9a1e5764\"},{\"content\":{\"connectorIds\":[\"Out3\"],\"side\":\"TOP\"},\"type\":\"ConnectorPlacement.EquallySpacedRectSide\",\"uuid\":\"9ba30cdf-1c12-4298-a5cc-99133179c3f0\"}]},\"type\":\"ConnectorPlacement.EquallySpacedConnector\",\"uuid\":\"81f0add0-9466-4071-a0a0-1fbb18cbe180\"}],\"packageUris\":[\"http://schema.mathworks.com/mf0/Connector/R2020b\"],\"version\":\"1.0\"}"
  Out1 : Outport
  Out2 : Outport  Port=2
  wires:
  state/1 -> Demux/1
  Demux/1 -> Trajectory Conversion - Point B1/1(x)
  Demux/2 -> Trajectory Conversion - Point B1/2(y)
  Demux/3 -> Trajectory Conversion - Point B1/3(theta)
  Trajectory Conversion - To Point B/1(d_xb) -> Mux2/1
  Trajectory Conversion - To Point B/2(d_yb) -> Mux2/2
  Mux2/1 -> Derivative/1, Sum/1
  Constant/1 -> MATLAB Function/2(b)
  Trajectory Conversion - Point B1/2(thetab) -> Trajectory Conversion - To Point B/3(theta), MATLAB Function/3(theta)
  Trajectory Generation/1(desired_x) -> Trajectory Conversion - To Point B/1(d_x)
  Trajectory Generation/2(desired_y) -> Trajectory Conversion - To Point B/2(d_y)
  Sum/1 -> Subsystem/1(In1)
  Derivative/1 -> Subsystem/2(In2)
  Subsystem/1(pb_dot) -> MATLAB Function/1(pb_dot)
  Trajectory Conversion - Point B1/1("xb, yb") -> Sum/2
  MATLAB Function/1(v) -> Mux1/1
  MATLAB Function/2(w) -> Mux1/2
  Mux1/1 -> Out1/1
  Trajectory Generation/3(Out1) -> Out2/1

== system unicycle/Unicycle Trajectory Tracking via Output Feedback CHAIN form - 1 ==
  state : Inport
  Demux : Demux  Outputs=3
  Integrator : Integrator
  Inverse Input Transform : Subsystem
  Mux : Mux  Inputs=2
  PD Controller : Subsystem
      settings: PortSchema="{\"entries\":[{\"content\":{\"sides\":[{\"content\":{\"connectorIds\":[\"In1\"]},\"type\":\"ConnectorPlacement.EquallySpacedRectSide\",\"uuid\":\"55bf99ca-bf04-473b-8ad6-9178bfa9531c\"},{\"content\":{\"connectorIds\":[\"Out1\"],\"side\":\"RIGHT\"},\"type\":\"ConnectorPlacement.EquallySpacedRectSide\",\"uuid\":\"b0ca0cd6-2a6e-4bef-9c4e-2c4670ff5894\"},{\"content\":{\"connectorIds\":[\"In2\"],\"side\":\"TOP\"},\"type\":\"ConnectorPlacement.EquallySpacedRectSide\",\"uuid\":\"e96b6c80-bb25-4e2c-8bad-15410e74167e\"}]},\"type\":\"ConnectorPlacement.EquallySpacedConnector\",\"uuid\":\"4638b46a-d87f-4eb7-bee0-6d662fc14ec0\"}],\"packageUris\":[\"http://schema.mathworks.com/mf0/Connector/R2020b\"],\"version\":\"1.0\"}"
  Sum : Sum  Inputs=|+-
  To State Z : Subsystem
  Trajectory Generation : Subsystem
      settings: PortSchema="{\"entries\":[{\"content\":{\"sides\":[{\"content\":{},\"type\":\"ConnectorPlacement.EquallySpacedRectSide\",\"uuid\":\"a0648d0c-83e2-4d86-998c-15587bd2a8bf\"},{\"content\":{\"connectorIds\":[\"Out1\"],\"side\":\"RIGHT\"},\"type\":\"ConnectorPlacement.EquallySpacedRectSide\",\"uuid\":\"9fd4a5b0-b008-42bf-83da-9f9a2612716d\"},{\"content\":{\"connectorIds\":[\"Out2\",\"Out3\"],\"side\":\"TOP\"},\"type\":\"ConnectorPlacement.EquallySpacedRectSide\",\"uuid\":\"29ce7ca0-3946-480f-b9bc-d0a41ca4b745\"}]},\"type\":\"ConnectorPlacement.EquallySpacedConnector\",\"uuid\":\"f091a176-3ac5-4616-b37c-ce46a3754a72\"}],\"packageUris\":[\"http://schema.mathworks.com/mf0/Connector/R2020b\"],\"version\":\"1.0\"}"
  v ,w : Outport
  Out1 : Outport  Port=2
  wires:
  Mux/1 -> v ,w/1
  state/1 -> Demux/1
  Demux/1 -> To State Z/1(x)
  Demux/2 -> To State Z/2(y)
  To State Z/1(z) -> Sum/2
  Sum/1 -> PD Controller/1(e)
  Integrator/1 -> Inverse Input Transform/3(v), Mux/1  "v"
  Trajectory Generation/1(z) -> Sum/1
  Trajectory Generation/2(z_dot) -> PD Controller/2(d_z_dot)  "Feedforward"
  Inverse Input Transform/1(a) -> Integrator/1
  PD Controller/1(u) -> Inverse Input Transform/1(u)
  Demux/3 -> Inverse Input Transform/2(theta)
  Inverse Input Transform/2(w) -> Mux/2
  Trajectory Generation/3(Out1) -> Out1/1

== system unicycle/Unicycle Trajectory Tracking via Output Feedback CHAIN form - 2 ==
  state : Inport
  Demux : Demux  Outputs=3
  Integrator : Integrator
  Inverse Input Transform : Subsystem
  Mux : Mux  Inputs=2
  PD Controller : Subsystem
      settings: PortSchema="{\"entries\":[{\"content\":{\"sides\":[{\"content\":{\"connectorIds\":[\"In1\"]},\"type\":\"ConnectorPlacement.EquallySpacedRectSide\",\"uuid\":\"55bf99ca-bf04-473b-8ad6-9178bfa9531c\"},{\"content\":{\"connectorIds\":[\"Out1\"],\"side\":\"RIGHT\"},\"type\":\"ConnectorPlacement.EquallySpacedRectSide\",\"uuid\":\"b0ca0cd6-2a6e-4bef-9c4e-2c4670ff5894\"},{\"content\":{\"connectorIds\":[\"In2\"],\"side\":\"TOP\"},\"type\":\"ConnectorPlacement.EquallySpacedRectSide\",\"uuid\":\"e96b6c80-bb25-4e2c-8bad-15410e74167e\"}]},\"type\":\"ConnectorPlacement.EquallySpacedConnector\",\"uuid\":\"4638b46a-d87f-4eb7-bee0-6d662fc14ec0\"}],\"packageUris\":[\"http://schema.mathworks.com/mf0/Connector/R2020b\"],\"version\":\"1.0\"}"
  Sum : Sum  Inputs=|+-
  To State Z : Subsystem
  Trajectory Generation : Subsystem
      settings: PortSchema="{\"entries\":[{\"content\":{\"sides\":[{\"content\":{},\"type\":\"ConnectorPlacement.EquallySpacedRectSide\",\"uuid\":\"a0648d0c-83e2-4d86-998c-15587bd2a8bf\"},{\"content\":{\"connectorIds\":[\"Out1\"],\"side\":\"RIGHT\"},\"type\":\"ConnectorPlacement.EquallySpacedRectSide\",\"uuid\":\"9fd4a5b0-b008-42bf-83da-9f9a2612716d\"},{\"content\":{\"connectorIds\":[\"Out2\",\"Out3\"],\"side\":\"TOP\"},\"type\":\"ConnectorPlacement.EquallySpacedRectSide\",\"uuid\":\"29ce7ca0-3946-480f-b9bc-d0a41ca4b745\"}]},\"type\":\"ConnectorPlacement.EquallySpacedConnector\",\"uuid\":\"f091a176-3ac5-4616-b37c-ce46a3754a72\"}],\"packageUris\":[\"http://schema.mathworks.com/mf0/Connector/R2020b\"],\"version\":\"1.0\"}"
  v ,w : Outport
  Out1 : Outport  Port=2
  wires:
  Mux/1 -> v ,w/1
  state/1 -> Demux/1
  Demux/1 -> To State Z/1(x)
  Demux/2 -> To State Z/2(y)
  To State Z/1(z) -> Sum/2
  Sum/1 -> PD Controller/1(e)
  Integrator/1 -> Inverse Input Transform/3(v), Mux/1  "v"
  Trajectory Generation/1(z) -> Sum/1
  Trajectory Generation/2(z_dot) -> PD Controller/2(d_z_dot)  "Feedforward"
  Inverse Input Transform/1(a) -> Integrator/1
  PD Controller/1(u) -> Inverse Input Transform/1(u)
  Demux/3 -> Inverse Input Transform/2(theta)
  Inverse Input Transform/2(w) -> Mux/2
  Trajectory Generation/3(Out1) -> Out1/1

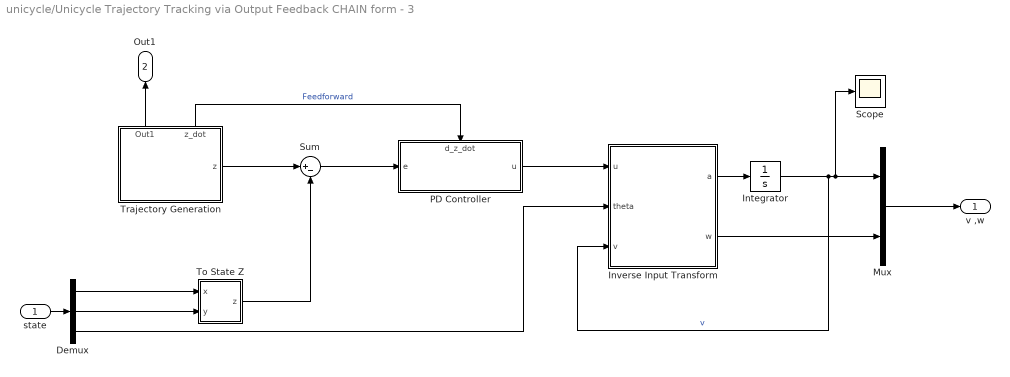
== system unicycle/Unicycle Trajectory Tracking via Output Feedback CHAIN form - 3 ==
  state : Inport
  Demux : Demux  Outputs=3
  Integrator : Integrator
  Inverse Input Transform : Subsystem
  Mux : Mux  Inputs=2
  PD Controller : Subsystem
      settings: PortSchema="{\"entries\":[{\"content\":{\"sides\":[{\"content\":{\"connectorIds\":[\"In1\"]},\"type\":\"ConnectorPlacement.EquallySpacedRectSide\",\"uuid\":\"55bf99ca-bf04-473b-8ad6-9178bfa9531c\"},{\"content\":{\"connectorIds\":[\"Out1\"],\"side\":\"RIGHT\"},\"type\":\"ConnectorPlacement.EquallySpacedRectSide\",\"uuid\":\"b0ca0cd6-2a6e-4bef-9c4e-2c4670ff5894\"},{\"content\":{\"connectorIds\":[\"In2\"],\"side\":\"TOP\"},\"type\":\"ConnectorPlacement.EquallySpacedRectSide\",\"uuid\":\"e96b6c80-bb25-4e2c-8bad-15410e74167e\"}]},\"type\":\"ConnectorPlacement.EquallySpacedConnector\",\"uuid\":\"4638b46a-d87f-4eb7-bee0-6d662fc14ec0\"}],\"packageUris\":[\"http://schema.mathworks.com/mf0/Connector/R2020b\"],\"version\":\"1.0\"}"
  Scope : Scope
  Sum : Sum  Inputs=|+-
  To State Z : Subsystem
  Trajectory Generation : Subsystem
      settings: PortSchema="{\"entries\":[{\"content\":{\"sides\":[{\"content\":{},\"type\":\"ConnectorPlacement.EquallySpacedRectSide\",\"uuid\":\"a0648d0c-83e2-4d86-998c-15587bd2a8bf\"},{\"content\":{\"connectorIds\":[\"Out1\"],\"side\":\"RIGHT\"},\"type\":\"ConnectorPlacement.EquallySpacedRectSide\",\"uuid\":\"9fd4a5b0-b008-42bf-83da-9f9a2612716d\"},{\"content\":{\"connectorIds\":[\"Out2\",\"Out3\"],\"side\":\"TOP\"},\"type\":\"ConnectorPlacement.EquallySpacedRectSide\",\"uuid\":\"29ce7ca0-3946-480f-b9bc-d0a41ca4b745\"}]},\"type\":\"ConnectorPlacement.EquallySpacedConnector\",\"uuid\":\"f091a176-3ac5-4616-b37c-ce46a3754a72\"}],\"packageUris\":[\"http://schema.mathworks.com/mf0/Connector/R2020b\"],\"version\":\"1.0\"}"
  v ,w : Outport
  Out1 : Outport  Port=2
  wires:
  Mux/1 -> v ,w/1
  state/1 -> Demux/1
  Demux/1 -> To State Z/1(x)
  Demux/2 -> To State Z/2(y)
  To State Z/1(z) -> Sum/2
  Sum/1 -> PD Controller/1(e)
  Integrator/1 -> Inverse Input Transform/3(v), Scope/1, Mux/1  "v"
  Trajectory Generation/1(z) -> Sum/1
  Trajectory Generation/3(z_dot) -> PD Controller/2(d_z_dot)  "Feedforward"
  Inverse Input Transform/1(a) -> Integrator/1
  PD Controller/1(u) -> Inverse Input Transform/1(u)
  Demux/3 -> Inverse Input Transform/2(theta)
  Inverse Input Transform/2(w) -> Mux/2
  Trajectory Generation/2(Out1) -> Out1/1

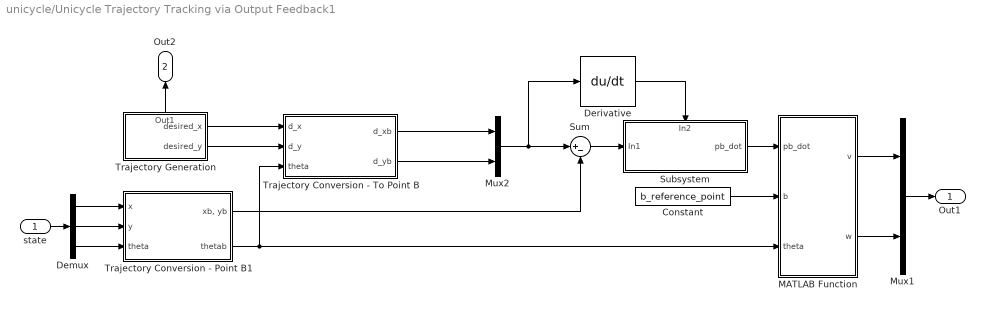
== system unicycle/Unicycle Trajectory Tracking via Output Feedback1 ==
  state : Inport
  Constant : Constant  Value=b_reference_point
  Demux : Demux  Outputs=3
  Derivative : Derivative
  MATLAB Function : MATLAB Function  TreatAsAtomicUnit=on
  Mux1 : Mux  Inputs=2
  Mux2 : Mux  Inputs=2
  Subsystem : Subsystem
      settings: PortSchema="{\"entries\":[{\"content\":{\"sides\":[{\"content\":{\"connectorIds\":[\"In1\"]},\"type\":\"ConnectorPlacement.EquallySpacedRectSide\",\"uuid\":\"e1edc101-a826-4003-ad08-df84a6d82578\"},{\"content\":{\"connectorIds\":[\"Out1\"],\"side\":\"RIGHT\"},\"type\":\"ConnectorPlacement.EquallySpacedRectSide\",\"uuid\":\"f1ed9078-3db7-4a0b-b785-0b08f9ba65fc\"},{\"content\":{\"connectorIds\":[\"In2\"],\"side\":\"TOP\"},\"type\":\"ConnectorPlacement.EquallySpacedRectSide\",\"uuid\":\"e7fa8122-daf7-4fc2-869b-ae0dcfffd8f2\"}]},\"type\":\"ConnectorPlacement.EquallySpacedConnector\",\"uuid\":\"a8720b8b-968d-49c2-bed5-00f70d36dfc2\"}],\"packageUris\":[\"http://schema.mathworks.com/mf0/Connector/R2020b\"],\"version\":\"1.0\"}"
  Sum : Sum  Inputs=|+-
  Trajectory Conversion - Point B1 : Subsystem
  Trajectory Conversion - To Point B : Subsystem
  Trajectory Generation : Subsystem
      settings: PortSchema="{\"entries\":[{\"content\":{\"sides\":[{\"content\":{},\"type\":\"ConnectorPlacement.EquallySpacedRectSide\",\"uuid\":\"27f935c9-4c91-4862-b00f-49430b536ba0\"},{\"content\":{\"connectorIds\":[\"Out1\",\"Out2\"],\"side\":\"RIGHT\"},\"type\":\"ConnectorPlacement.EquallySpacedRectSide\",\"uuid\":\"fd268e79-917c-4566-a618-4e3d9a1e5764\"},{\"content\":{\"connectorIds\":[\"Out3\"],\"side\":\"TOP\"},\"type\":\"ConnectorPlacement.EquallySpacedRectSide\",\"uuid\":\"9ba30cdf-1c12-4298-a5cc-99133179c3f0\"}]},\"type\":\"ConnectorPlacement.EquallySpacedConnector\",\"uuid\":\"81f0add0-9466-4071-a0a0-1fbb18cbe180\"}],\"packageUris\":[\"http://schema.mathworks.com/mf0/Connector/R2020b\"],\"version\":\"1.0\"}"
  Out1 : Outport
  Out2 : Outport  Port=2
  wires:
  state/1 -> Demux/1
  Demux/1 -> Trajectory Conversion - Point B1/1(x)
  Demux/2 -> Trajectory Conversion - Point B1/2(y)
  Demux/3 -> Trajectory Conversion - Point B1/3(theta)
  Trajectory Conversion - To Point B/1(d_xb) -> Mux2/1
  Trajectory Conversion - To Point B/2(d_yb) -> Mux2/2
  Mux2/1 -> Derivative/1, Sum/1
  Constant/1 -> MATLAB Function/2(b)
  Trajectory Conversion - Point B1/2(thetab) -> Trajectory Conversion - To Point B/3(theta), MATLAB Function/3(theta)
  Trajectory Generation/1(desired_x) -> Trajectory Conversion - To Point B/1(d_x)
  Trajectory Generation/2(desired_y) -> Trajectory Conversion - To Point B/2(d_y)
  Sum/1 -> Subsystem/1(In1)
  Derivative/1 -> Subsystem/2(In2)
  Subsystem/1(pb_dot) -> MATLAB Function/1(pb_dot)
  Trajectory Conversion - Point B1/1("xb, yb") -> Sum/2
  MATLAB Function/1(v) -> Mux1/1
  MATLAB Function/2(w) -> Mux1/2
  Mux1/1 -> Out1/1
  Trajectory Generation/3(Out1) -> Out2/1

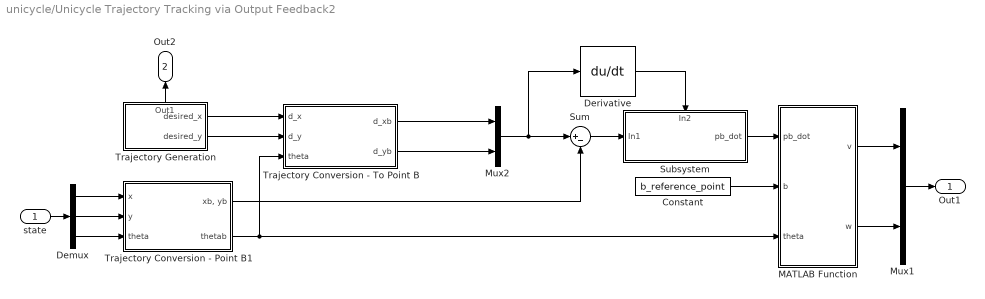
== system unicycle/Unicycle Trajectory Tracking via Output Feedback2 ==
  state : Inport
  Constant : Constant  Value=b_reference_point
  Demux : Demux  Outputs=3
  Derivative : Derivative
  MATLAB Function : MATLAB Function  TreatAsAtomicUnit=on
  Mux1 : Mux  Inputs=2
  Mux2 : Mux  Inputs=2
  Subsystem : Subsystem
      settings: PortSchema="{\"entries\":[{\"content\":{\"sides\":[{\"content\":{\"connectorIds\":[\"In1\"]},\"type\":\"ConnectorPlacement.EquallySpacedRectSide\",\"uuid\":\"e1edc101-a826-4003-ad08-df84a6d82578\"},{\"content\":{\"connectorIds\":[\"Out1\"],\"side\":\"RIGHT\"},\"type\":\"ConnectorPlacement.EquallySpacedRectSide\",\"uuid\":\"f1ed9078-3db7-4a0b-b785-0b08f9ba65fc\"},{\"content\":{\"connectorIds\":[\"In2\"],\"side\":\"TOP\"},\"type\":\"ConnectorPlacement.EquallySpacedRectSide\",\"uuid\":\"e7fa8122-daf7-4fc2-869b-ae0dcfffd8f2\"}]},\"type\":\"ConnectorPlacement.EquallySpacedConnector\",\"uuid\":\"a8720b8b-968d-49c2-bed5-00f70d36dfc2\"}],\"packageUris\":[\"http://schema.mathworks.com/mf0/Connector/R2020b\"],\"version\":\"1.0\"}"
  Sum : Sum  Inputs=|+-
  Trajectory Conversion - Point B1 : Subsystem
  Trajectory Conversion - To Point B : Subsystem
  Trajectory Generation : Subsystem
      settings: PortSchema="{\"entries\":[{\"content\":{\"sides\":[{\"content\":{},\"type\":\"ConnectorPlacement.EquallySpacedRectSide\",\"uuid\":\"8d5b539f-cb35-429e-a5fa-cedc5caa952f\"},{\"content\":{\"connectorIds\":[\"Out1\",\"Out2\"],\"side\":\"RIGHT\"},\"type\":\"ConnectorPlacement.EquallySpacedRectSide\",\"uuid\":\"95bf0b02-bf52-4ab7-8c48-02064be9b571\"},{\"content\":{\"connectorIds\":[\"Out3\"],\"side\":\"TOP\"},\"type\":\"ConnectorPlacement.EquallySpacedRectSide\",\"uuid\":\"a2bfc8c2-4d82-41c7-adad-fabfe4183f1a\"}]},\"type\":\"ConnectorPlacement.EquallySpacedConnector\",\"uuid\":\"366492ce-5a31-4dd6-b5f7-03158cf0c801\"}],\"packageUris\":[\"http://schema.mathworks.com/mf0/Connector/R2020b\"],\"version\":\"1.0\"}"
  Out1 : Outport
  Out2 : Outport  Port=2
  wires:
  state/1 -> Demux/1
  Demux/1 -> Trajectory Conversion - Point B1/1(x)
  Demux/2 -> Trajectory Conversion - Point B1/2(y)
  Demux/3 -> Trajectory Conversion - Point B1/3(theta)
  Trajectory Conversion - To Point B/1(d_xb) -> Mux2/1
  Trajectory Conversion - To Point B/2(d_yb) -> Mux2/2
  Mux2/1 -> Derivative/1, Sum/1
  Constant/1 -> MATLAB Function/2(b)
  Trajectory Conversion - Point B1/2(thetab) -> Trajectory Conversion - To Point B/3(theta), MATLAB Function/3(theta)
  Trajectory Generation/1(desired_x) -> Trajectory Conversion - To Point B/1(d_x)
  Trajectory Generation/2(desired_y) -> Trajectory Conversion - To Point B/2(d_y)
  Sum/1 -> Subsystem/1(In1)
  Derivative/1 -> Subsystem/2(In2)
  Subsystem/1(pb_dot) -> MATLAB Function/1(pb_dot)
  Trajectory Conversion - Point B1/1("xb, yb") -> Sum/2
  MATLAB Function/1(v) -> Mux1/1
  MATLAB Function/2(w) -> Mux1/2
  Mux1/1 -> Out1/1
  Trajectory Generation/3(Out1) -> Out2/1

== system unicycle/Controller Switching/Boolean Logic ==
  e : Inport
  "Compute the distance " : MATLAB Function  TreatAsAtomicUnit=on
  Constant : Constant  Value=0
  If : If  IfExpression=u1 <= rv_distance
  If Action Subsystem : Subsystem  TreatAsAtomicUnit=on
  If Action Subsystem1 : Subsystem  TreatAsAtomicUnit=on
  Scope : Scope
  Sum : Sum
  Out1 : Outport
  e_l : Outport  Port=2
  wires:
  Sum/1 -> Out1/1, Scope/1
  If/1 -> If Action Subsystem/Action
  "Compute the distance "/1(e_l) -> If/1, e_l/1
  If Action Subsystem/1(Out1) -> Sum/1
  If/2 -> If Action Subsystem1/Action
  If Action Subsystem1/1(Out1) -> Sum/2
  e/1 -> "Compute the distance "/1(e)
  Constant/1 -> If Action Subsystem1/1(In1), If Action Subsystem/1(In1)

== system unicycle/Controller Switching  /Boolean Logic ==
  e : Inport
  "Compute the distance " : MATLAB Function  TreatAsAtomicUnit=on
  Constant : Constant  Value=0
  If : If  IfExpression=u1 <= rv_distance
  If Action Subsystem : Subsystem  TreatAsAtomicUnit=on
  If Action Subsystem1 : Subsystem  TreatAsAtomicUnit=on
  Scope : Scope
  Sum : Sum  Inputs=|++
  Out1 : Outport
  e_l : Outport  Port=2
  wires:
  Sum/1 -> Out1/1, Scope/1
  If/1 -> If Action Subsystem/Action
  "Compute the distance "/1(e_l) -> e_l/1, If/1
  If Action Subsystem/1(Out1) -> Sum/1
  If/2 -> If Action Subsystem1/Action
  Constant/1 -> If Action Subsystem1/1(In1), If Action Subsystem/1(In1)
  If Action Subsystem1/1(Out1) -> Sum/2
  e/1 -> "Compute the distance "/1(e)

== system unicycle/Controller Switching2/Boolean Logic ==
  e : Inport
  "Compute the distance " : MATLAB Function  TreatAsAtomicUnit=on
  Constant : Constant  Value=0
  If : If  IfExpression=u1 <= rv_distance
  If Action Subsystem : Subsystem  TreatAsAtomicUnit=on
  If Action Subsystem1 : Subsystem  TreatAsAtomicUnit=on
  Scope : Scope
  Sum : Sum  Inputs=|++
  Out1 : Outport
  e_l : Outport  Port=2
  wires:
  Sum/1 -> Out1/1, Scope/1
  If/1 -> If Action Subsystem/Action
  "Compute the distance "/1(e_l) -> If/1, e_l/1
  If Action Subsystem/1(Out1) -> Sum/1
  If/2 -> If Action Subsystem1/Action
  Constant/1 -> If Action Subsystem1/1(In1), If Action Subsystem/1(In1)
  If Action Subsystem1/1(Out1) -> Sum/2
  e/1 -> "Compute the distance "/1(e)
